simulink model "untitled"  (R2024b)
settings: Solver=VariableStepAuto  StartTime=0.0  StopTime=1  RelTol=1e-3
libraries: spsMosfetLib x14, spsSeriesRLCBranchLib x11, spsDCVoltageSourceLib x5, simulink x5, spsVoltageMeasurementLib x5, spsIdealSwitchLib x2, spsThreePhaseSeriesRLCBranchLib x2, spsCurrentMeasurementLib x1, spsDiodeLib x1, spsLinearTransformerLib x1, spspowerguiLib x1
settings Model: LastModifiedBy=dsz

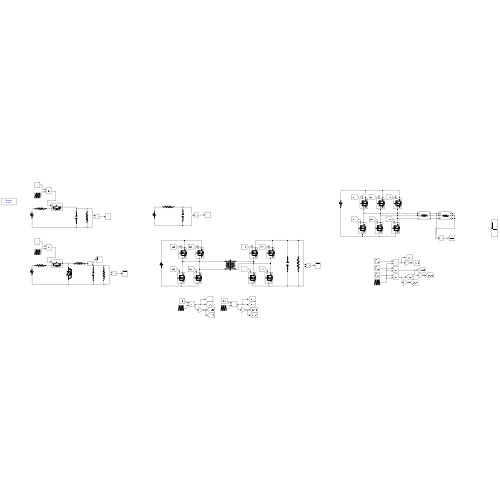
[thumbnail: Simulink's stored preview of the top-level diagram]
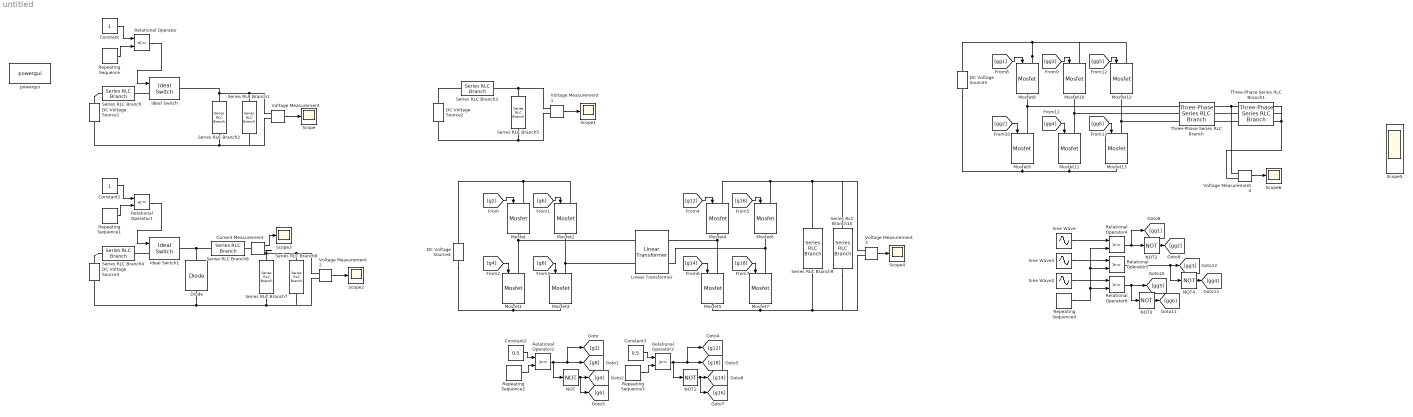
== system untitled ==
  Constant : Constant
  Constant1 : Constant
  Constant2 : Constant  Value=0.5
  Constant3 : Constant  Value=0.5
  Current Measurement : spsCurrentMeasurementLib/Current Measurement  PhasorSimulation=off  OutputType=Complex  PSBequivalent=0
  DC Voltage Source{1..3,5} (4 alike) : spsDCVoltageSourceLib/DC Voltage Source  Amplitude=100  Measurements=None
  DC Voltage Source4 : spsDCVoltageSourceLib/DC Voltage Source  Amplitude=200  Measurements=None
  Diode : spsDiodeLib/Diode  Ron=0.001  Lon=0  Vf=0  IC=0  UseSnubber=0  Rs=500  Cs=250e-9  Measurements=off
  Ideal Switch : spsIdealSwitchLib/Ideal Switch  Ron=0.001  Lon=0  IC=1  Rs=1e5  Cs=inf  Measurements=off
  Ideal Switch1 : spsIdealSwitchLib/Ideal Switch  Ron=0.001  Lon=0  IC=1  Rs=1e5  Cs=inf  Measurements=off
  Linear Transformer : spsLinearTransformerLib/Linear Transformer  UNITS=SI  NominalPower=[ 250e6 1000 ]  winding1=[200 0 0]  winding2=[400 0 0]  ThreeWindings=off  winding3=[3.15e+05 0.7938 0.084225]  RmLm=[0 1e-4]  Measurements=None  DataType=on
  Mosfet{,1..13} (14 alike) : spsMosfetLib/Mosfet  Ron=0.01  Lon=0  Rd=0.01  Vfd=0  IC=0  Rs=1e5  Cs=inf  Measurements=off
  NOT{,1..4} (5 alike) : Logic  Operator=NOT  IconShape=distinctive  AllPortsSameDT=off  OutDataTypeStr=boolean
  Relational Operator : RelationalOperator  Operator=<=  OutDataTypeStr=boolean  RndMeth=Simplest  InputSameDT=off
  Relational Operator1 : RelationalOperator  Operator=<=  OutDataTypeStr=boolean  RndMeth=Simplest  InputSameDT=off
  Relational Operator{2..6} (5 alike) : RelationalOperator  OutDataTypeStr=boolean  RndMeth=Simplest  InputSameDT=off
  Repeating Sequence : simulink/Sources/Repeating Sequence  rep_seq_t=[0 0.002]  rep_seq_y=[0 2]
  Repeating Sequence1 : simulink/Sources/Repeating Sequence  rep_seq_t=[0 0.002]  rep_seq_y=[0 2]
  Repeating Sequence2 : simulink/Sources/Repeating Sequence  rep_seq_t=[0 5e-4 1e-3]  rep_seq_y=[0 1 0]
  Repeating Sequence3 : simulink/Sources/Repeating Sequence  rep_seq_t=[1e-4 6e-4 11e-4]  rep_seq_y=[0 1 0]
  Repeating Sequence4 : simulink/Sources/Repeating Sequence  rep_seq_t=[0 5e-4 1e-3]  rep_seq_y=[0 1 0]
  Scope{,1..6} (7 alike) : Scope
  Series RLC Branch : spsSeriesRLCBranchLib/Series RLC Branch  LConnTagsString=__new0  RConnTagsString=__new0  BranchType=R  Resistance=1  Inductance=1e-3  SetiL0=off  InitialCurrent=0  Capacitance=1e-6  Setx0=off  InitialVoltage=0  Measurements=None
  Series RLC Branch1 : spsSeriesRLCBranchLib/Series RLC Branch  LConnTagsString=__new0  RConnTagsString=__new0  BranchType=R  Resistance=100  Inductance=1e-3  SetiL0=off  InitialCurrent=0  Capacitance=1e-6  Setx0=off  InitialVoltage=0  Measurements=None
  Series RLC Branch10 : spsSeriesRLCBranchLib/Series RLC Branch  LConnTagsString=__new0  RConnTagsString=__new0  BranchType=R  Resistance=30  Inductance=1e-3  SetiL0=off  InitialCurrent=0  Capacitance=1e-6  Setx0=off  InitialVoltage=0  Measurements=None
  Series RLC Branch2 : spsSeriesRLCBranchLib/Series RLC Branch  LConnTagsString=__new0  RConnTagsString=__new0  BranchType=C  Resistance=1  Inductance=1e-3  SetiL0=off  InitialCurrent=0  Capacitance=1e-3  Setx0=on  InitialVoltage=0  Measurements=None
  Series RLC Branch3 : spsSeriesRLCBranchLib/Series RLC Branch  LConnTagsString=__new0  RConnTagsString=__new0  BranchType=R  Resistance=1e3  Inductance=1e-3  SetiL0=off  InitialCurrent=0  Capacitance=1e-6  Setx0=off  InitialVoltage=0  Measurements=None
  Series RLC Branch4 : spsSeriesRLCBranchLib/Series RLC Branch  LConnTagsString=__new0  RConnTagsString=__new0  BranchType=R  Resistance=0.1  Inductance=1e-3  SetiL0=off  InitialCurrent=0  Capacitance=1e-6  Setx0=off  InitialVoltage=0  Measurements=None
  Series RLC Branch5 : spsSeriesRLCBranchLib/Series RLC Branch  LConnTagsString=__new0  RConnTagsString=__new0  BranchType=C  Resistance=1  Inductance=1e-3  SetiL0=off  InitialCurrent=0  Capacitance=1e-3  Setx0=on  InitialVoltage=0  Measurements=None
  Series RLC Branch6 : spsSeriesRLCBranchLib/Series RLC Branch  LConnTagsString=__new0  RConnTagsString=__new0  BranchType=R  Resistance=100  Inductance=1e-3  SetiL0=off  InitialCurrent=0  Capacitance=1e-6  Setx0=off  InitialVoltage=0  Measurements=None
  Series RLC Branch7 : spsSeriesRLCBranchLib/Series RLC Branch  LConnTagsString=__new0  RConnTagsString=__new0  BranchType=C  Resistance=1  Inductance=1e-3  SetiL0=off  InitialCurrent=0  Capacitance=1e-3  Setx0=on  InitialVoltage=0  Measurements=None
  Series RLC Branch8 : spsSeriesRLCBranchLib/Series RLC Branch  LConnTagsString=__new0  RConnTagsString=__new0  BranchType=L  Resistance=0.1  Inductance=1e-2  SetiL0=on  InitialCurrent=0  Capacitance=1e-6  Setx0=off  InitialVoltage=0  Measurements=None
  Series RLC Branch9 : spsSeriesRLCBranchLib/Series RLC Branch  LConnTagsString=__new0  RConnTagsString=__new0  BranchType=C  Resistance=1  Inductance=1e-3  SetiL0=off  InitialCurrent=0  Capacitance=680e-6  Setx0=off  InitialVoltage=0  Measurements=None
  Sine Wave : Sin  Amplitude=0.5  Frequency=50*2*pi  SampleTime=0
  Sine Wave1 : Sin  Amplitude=0.5  Frequency=50*2*pi  Phase=2/3*pi  SampleTime=0
  Sine Wave2 : Sin  Amplitude=0.5  Frequency=50*2*pi  Phase=4/3*pi  SampleTime=0
  Three-Phase Series RLC Branch : spsThreePhaseSeriesRLCBranchLib/Three-Phase Series RLC Branch  LConnTagsString=A|B|C  RConnTagsString=A|B|C  BranchType=L  Resistance=10  Inductance=0.1  Capacitance=1e-6  Measurements=Branch voltages and currents
  Three-Phase Series RLC Branch1 : spsThreePhaseSeriesRLCBranchLib/Three-Phase Series RLC Branch  LConnTagsString=A|B|C  RConnTagsString=A|B|C  BranchType=R  Resistance=10  Inductance=0.1  Capacitance=1e-6  Measurements=Branch voltages and currents
  Voltage Measurement{,1..4} (5 alike) : spsVoltageMeasurementLib/Voltage Measurement  PhasorSimulation=off  OutputType=Complex  PSBequivalent=0
  powergui : spspowerguiLib/powergui  Priority=1  SimulationMode=Discrete  SampleTime=1e-5  frequency=60  Iterations=50  frequencyindice=0  Pbase=100e6  ErrMax=1e-4  UnitsV=kV  UnitsW=MW  buscounter=0  FunctionMessages=off  echomessages=off  EnableUseOfTLC=off  CurrentSourceSwitches=off  DisableSnubberDevices=off  DisableRonSwitches=off  DisableVfSwitches=off  DisplayEquations=off  AutomaticDiscreteSolvers=off  SolverType=Tustin/Backward Euler (TBE)  Interpol=off  ExternalGateDelay=off  methode=off  Ts=100  x0status=blocks  SPID=on  SwTol=0  HookPort=off  NonlinearTolerance=1e-4  nMaxIteration=100  ContinueOnMaxIteration=off  RestoreLinks=warning  ResistiveCurrentMeasurement=off  Frange=[0:2:500]  Ylog=off  Xlog=on  ShowGrid=off  save=off  variable=ZData  structure=0  ZoomFFT=off  StartTime=0.0  cycles=1  DisplayStyle=1  fundamental=60  FreqAxis=off  MaxFrequency=1000  frequencyindicesteady=1  RmsSteady=1  display=off
  wires:
  Constant/1 -> Relational Operator/1
  Repeating Sequence/1 -> Relational Operator/2
  Relational Operator/1 -> Ideal Switch/1
  Voltage Measurement/1 -> Scope/1
  Voltage Measurement1/1 -> Scope1/1
  Voltage Measurement2/1 -> Scope2/1
  Relational Operator1/1 -> Ideal Switch1/1
  Repeating Sequence1/1 -> Relational Operator1/2
  Constant1/1 -> Relational Operator1/1
  Current Measurement/1 -> Scope3/1
  [g2] -> Mosfet/1
  [g6] -> Mosfet2/1
  [g4] -> Mosfet1/1
  [g8] -> Mosfet3/1
  [g18] -> Mosfet7/1
  [g14] -> Mosfet5/1
  [g16] -> Mosfet6/1
  [g12] -> Mosfet4/1
  Constant2/1 -> Relational Operator2/1
  Repeating Sequence2/1 -> Relational Operator2/2
  Relational Operator2/1 -> NOT/1, [g8], [g2]
  NOT/1 -> [g6], [g4]
  NOT1/1 -> [g14], [g16]
  Relational Operator3/1 -> [g12], [g18], NOT1/1
  Repeating Sequence3/1 -> Relational Operator3/2
  Constant3/1 -> Relational Operator3/1
  Voltage Measurement3/1 -> Scope4/1
  [gg4] -> Mosfet11/1
  [gg2] -> Mosfet9/1
  [gg3] -> Mosfet10/1
  [gg1] -> Mosfet8/1
  [gg5] -> Mosfet12/1
  [gg6] -> Mosfet13/1
  Sine Wave/1 -> Relational Operator4/1
  Sine Wave1/1 -> Relational Operator5/1
  Sine Wave2/1 -> Relational Operator6/1
  Repeating Sequence4/1 -> Relational Operator6/2, Relational Operator5/2, Relational Operator4/2
  Relational Operator4/1 -> NOT2/1, [gg1]
  NOT2/1 -> [gg2]
  Relational Operator6/1 -> NOT3/1, [gg5]
  NOT3/1 -> [gg6]
  NOT4/1 -> [gg4]
  Relational Operator5/1 -> NOT4/1, [gg3]
  Voltage Measurement4/1 -> Scope6/1
  connections:
  DC Voltage Source1/RConn1 -- Series RLC Branch/LConn1
  Ideal Switch/LConn1 -- Series RLC Branch/RConn1
  Series RLC Branch2/LConn1 -- Voltage Measurement/LConn1 -- Series RLC Branch1/LConn1 -- Ideal Switch/RConn1
  Series RLC Branch2/RConn1 -- Voltage Measurement/LConn2 -- Series RLC Branch1/RConn1 -- DC Voltage Source1/LConn1
  Series RLC Branch5/RConn1 -- DC Voltage Source2/LConn1 -- Voltage Measurement1/LConn2
  DC Voltage Source2/RConn1 -- Series RLC Branch3/LConn1
  Series RLC Branch5/LConn1 -- Series RLC Branch3/RConn1 -- Voltage Measurement1/LConn1
  Series RLC Branch7/LConn1 -- Current Measurement/RConn1 -- Series RLC Branch6/LConn1 -- Voltage Measurement2/LConn1
  Series RLC Branch7/RConn1 -- DC Voltage Source3/LConn1 -- Diode/LConn1 -- Series RLC Branch6/RConn1 -- Voltage Measurement2/LConn2
  Ideal Switch1/LConn1 -- Series RLC Branch4/RConn1
  DC Voltage Source3/RConn1 -- Series RLC Branch4/LConn1
  Series RLC Branch8/LConn1 -- Ideal Switch1/RConn1 -- Diode/RConn1
  Current Measurement/LConn1 -- Series RLC Branch8/RConn1
  Mosfet1/LConn1 -- Linear Transformer/LConn1 -- Mosfet/RConn1
  Mosfet3/LConn1 -- Linear Transformer/LConn2 -- Mosfet2/RConn1
  DC Voltage Source4/RConn1 -- Mosfet/LConn1 -- Mosfet2/LConn1
  DC Voltage Source4/LConn1 -- Mosfet3/RConn1 -- Mosfet1/RConn1
  Mosfet5/LConn1 -- Linear Transformer/RConn1 -- Mosfet4/RConn1
  Mosfet7/LConn1 -- Linear Transformer/RConn2 -- Mosfet6/RConn1
  Mosfet6/LConn1 -- Series RLC Branch10/LConn1 -- Voltage Measurement3/LConn1 -- Series RLC Branch9/LConn1 -- Mosfet4/LConn1
  Mosfet7/RConn1 -- Series RLC Branch10/RConn1 -- Voltage Measurement3/LConn2 -- Series RLC Branch9/RConn1 -- Mosfet5/RConn1
  Mosfet9/LConn1 -- Three-Phase Series RLC Branch/LConn1 -- Mosfet8/RConn1
  Mosfet11/LConn1 -- Three-Phase Series RLC Branch/LConn2 -- Mosfet10/RConn1
  Mosfet8/LConn1 -- Mosfet12/LConn1 -- Mosfet10/LConn1 -- DC Voltage Source5/RConn1
  Mosfet13/LConn1 -- Three-Phase Series RLC Branch/LConn3 -- Mosfet12/RConn1
  Three-Phase Series RLC Branch1/LConn1 -- Voltage Measurement4/LConn1 -- Three-Phase Series RLC Branch/RConn1
  Three-Phase Series RLC Branch1/LConn3 -- Three-Phase Series RLC Branch/RConn3
  Three-Phase Series RLC Branch1/LConn2 -- Three-Phase Series RLC Branch/RConn2
  Mosfet13/RConn1 -- DC Voltage Source5/LConn1 -- Mosfet9/RConn1 -- Mosfet11/RConn1
  Three-Phase Series RLC Branch1/RConn1 -- Three-Phase Series RLC Branch1/RConn2 -- Three-Phase Series RLC Branch1/RConn3 -- Voltage Measurement4/LConn2
